simulink model "Simulator"  (R2024a)
settings: Solver=FixedStepAuto  StartTime=0.0  StopTime=1600  RelTol=1e-3
values from neighbouring files (symbols this model uses):
  T = loadturbineconstants('IEA15MW')    [init_controller.m]
  Wr0 = 0.60    (= 0.6)    [init_controller.m]
undefined symbols (not defined in the file or in its folder): DiscIntNeverNeededParam
libraries: DRC_SimulinkLibrary x3
settings Model: Creator=glazzerini  LastModifiedBy=glazzerini

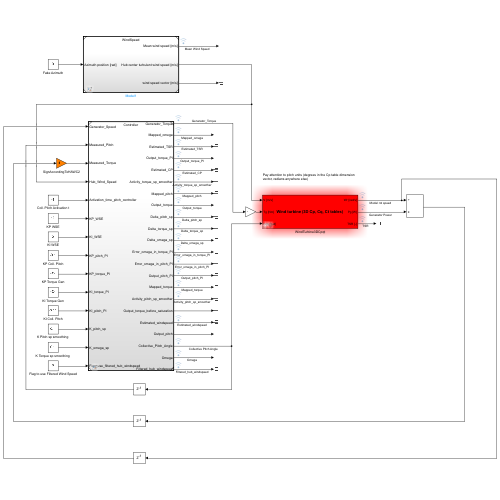
[thumbnail: Simulink's stored preview of the top-level diagram]
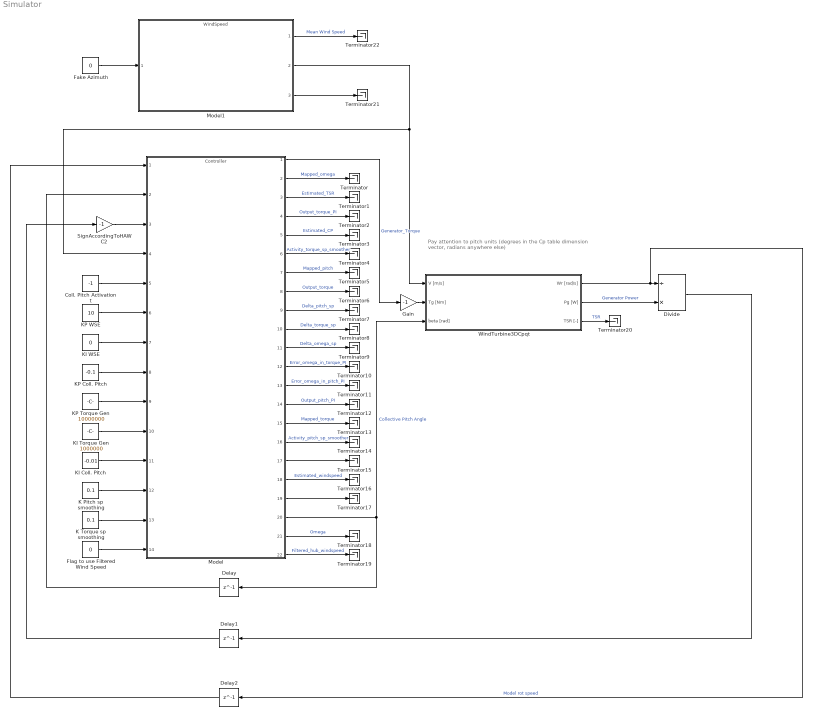
== system Simulator ==
  note: Pay attention to pitch units (degrees in the Cp table dimension vector, radians anywhere else)
  Coll. Pitch Activation t : Constant  Value=-1
  Delay : Delay  DelayLength=1
  Delay1 : Delay  DelayLength=1
  Delay2 : Delay  DelayLength=1
  Divide : Product  Inputs=/*
  Fake Azimuth : Constant  Value=0
  Flag to use Filtered Wind Speed : Constant  Value=0
  Gain : Gain  Gain=-1
  "K Pitch sp smoothing " : Constant  Value=0.1
  "K Torque sp smoothing " : Constant  Value=0.1
  KI Coll. Pitch : Constant  Value=-0.01
  KI Torque Gen : Constant  Value=1000000
  KI WSE : Constant  Value=0
  KP Coll. Pitch : Constant  Value=-0.1
  KP Torque Gen : Constant  Value=10000000
  KP WSE : Constant  Value=10
  Model : ModelReference  ModelNameDialog=Controller.slx  SimulationMode=Normal  ModelReferenceVersion=18.123
  Model1 : ModelReference  ModelNameDialog=WindSpeed.slx  SimulationMode=Normal  ModelReferenceVersion=9.19
  SignAccordingToHAWC2 : Gain  Gain=-1
  Terminator{,1..22} (23 alike) : Terminator
  WindTurbine3DCpqt : Subsystem  AncestorBlock=DRC_SimulinkLibrary/WindTurbine3DCpqt  mask{R=T.R, rho=T.rho, TMax=inf, JWr=T.Jlss, G=T.G, Wr0=Wr0, GenEfficiency=T.etag, CpArray=T.Cp, betaVec=deg2rad(T.CPitch), wsVec=T.CWindSpeed, omegaVec=T.COmega}
      mask prompts: R "Rotor radius [m]"; rho "Air density [kg/m^3]"; TMax "Maximum aerodynamic torque [Nm]"; JWr "Inertia low-speed shaft [kg m^2]"; G "Gearbox ratio [-]"; Wr0 "Rotor speed initial condition [rad/s]"; GenEfficiency "Generator Efficiency [-]"; CpArray "Cp matrix"; betaVec "Pitch vector [rad]"; wsVec "Wind speed vector [m/s]"; omegaVec "Omega vector [rad/s]"
      mask DialogControl CpGroupVar Prompt: Power coefficient (Cp)
      mask Display: disp('{\bf\fontsize{12}Wind turbine (3D Cp, Cq, Ct tables)}', 'texmode', 'on');
  wires:
  Model/1 -> Gain/1  "Generator_Torque"
  Model/20 -> WindTurbine3DCpqt/3(beta [rad]), Delay/1  "Collective Pitch Angle"
  WindTurbine3DCpqt/1(Wr [rad/s]) -> Divide/1, Delay2/1  "Model rot speed"
  Model/2 -> Terminator/1  "Mapped_omega"
  Model/3 -> Terminator1/1  "Estimated_TSR"
  Model/4 -> Terminator2/1  "Output_torque_PI"
  Model/5 -> Terminator3/1  "Estimated_CP"
  Model/6 -> Terminator4/1  "Activity_torque_sp_smoother"
  Model/7 -> Terminator5/1  "Mapped_pitch"
  Model/8 -> Terminator6/1  "Output_torque"
  Model/9 -> Terminator7/1  "Delta_pitch_sp"
  Model/10 -> Terminator8/1  "Delta_torque_sp"
  Model/11 -> Terminator9/1  "Delta_omega_sp"
  Model/12 -> Terminator10/1  "Error_omega_in_torque_PI"
  Model/13 -> Terminator11/1  "Error_omega_in_pitch_PI"
  Model/14 -> Terminator12/1  "Output_pitch_PI"
  Model/15 -> Terminator13/1  "Mapped_torque"
  Model/16 -> Terminator14/1  "Activity_pitch_sp_smoother"
  Model/17 -> Terminator15/1
  Model/18 -> Terminator16/1  "Estimated_windspeed"
  Model/19 -> Terminator17/1
  Model/21 -> Terminator18/1  "Omega"
  Model/22 -> Terminator19/1  "Filtered_hub_windspeed"
  Delay/1 -> Model/2
  WindTurbine3DCpqt/3(TSR [-]) -> Terminator20/1  "TSR"
  WindTurbine3DCpqt/2(Pg [W]) -> Divide/2  "Generator Power"
  Divide/1 -> Delay1/1
  Delay1/1 -> SignAccordingToHAWC2/1
  "K Torque sp smoothing "/1 -> Model/13
  "K Pitch sp smoothing "/1 -> Model/12
  Coll. Pitch Activation t/1 -> Model/5
  KP Torque Gen/1 -> Model/9
  KI Torque Gen/1 -> Model/10
  KP Coll. Pitch/1 -> Model/8
  KI Coll. Pitch/1 -> Model/11
  KP WSE/1 -> Model/6
  KI WSE/1 -> Model/7
  Model1/2 -> Model/4, WindTurbine3DCpqt/1(V [m/s])
  Fake Azimuth/1 -> Model1/1
  Model1/3 -> Terminator21/1
  Model1/1 -> Terminator22/1  "Mean Wind Speed"
  Gain/1 -> WindTurbine3DCpqt/2(Tg [Nm])
  Delay2/1 -> Model/1
  SignAccordingToHAWC2/1 -> Model/3
  Flag to use Filtered Wind Speed/1 -> Model/14

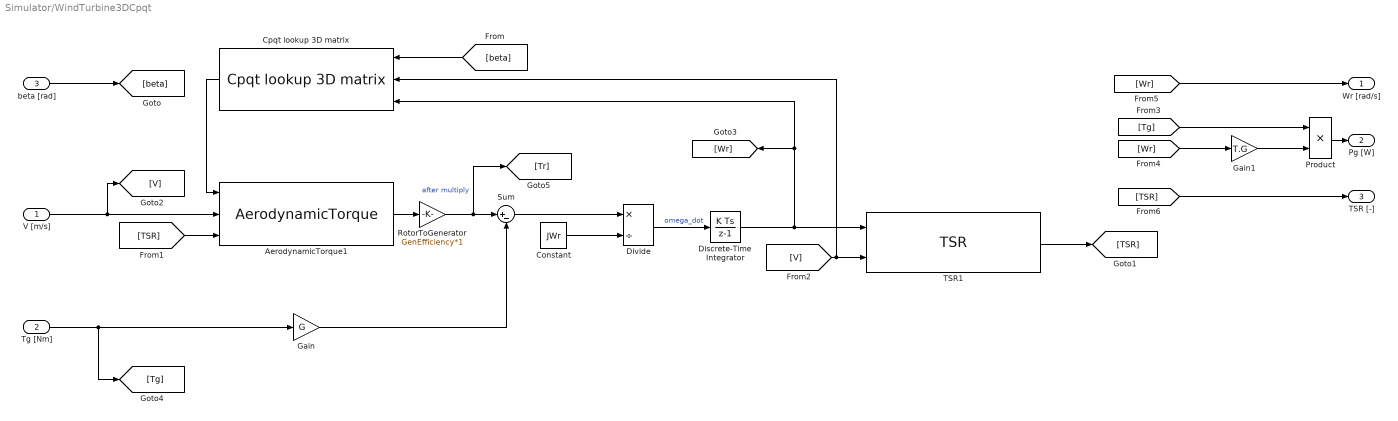
== system Simulator/WindTurbine3DCpqt ==
  V [m/s] : Inport
  Tg [Nm] : Inport  Port=2
  beta [rad] : Inport  Port=3
  AerodynamicTorque1 : DRC_SimulinkLibrary/AerodynamicTorque  R=R  rho=rho  TrMax=TMax
  Constant : Constant  Value=JWr
  Cpqt lookup 3D matrix : DRC_SimulinkLibrary/Cpqt lookup 3D matrix  CpqtGrid=CpArray  PitchVector=betaVec  WindSpeedVector=wsVec  OmegaVector=omegaVec
  Discrete-Time Integrator : DiscreteIntegrator  InitialCondition=Wr0  SampleTime=-1  ICPrevOutput=DiscIntNeverNeededParam  ICPrevScaledInput=DiscIntNeverNeededParam
  Divide : Product  Inputs=*/
  Gain : Gain  Gain=G
  Gain1 : Gain  Gain=T.G
  Product : Product
  RotorToGenerator : Gain  Gain=GenEfficiency*1
  Sum : Sum  Inputs=|+-
  TSR1 : DRC_SimulinkLibrary/TSR  RotorRadius=R
  Wr [rad/s] : Outport
  Pg [W] : Outport  Port=2
  TSR [-] : Outport  Port=3
  wires:
  Cpqt lookup 3D matrix/1 -> AerodynamicTorque1/1
  [TSR] -> TSR [-]/1
  [Wr] -> Wr [rad/s]/1
  [Tg] -> Product/1
  [Wr] -> Gain1/1
  Product/1 -> Pg [W]/1
  Gain1/1 -> Product/2
  [V] -> TSR1/2, Cpqt lookup 3D matrix/2
  TSR1/1 -> [TSR]
  Sum/1 -> Divide/1
  AerodynamicTorque1/1 -> RotorToGenerator/1
  Discrete-Time Integrator/1 -> TSR1/1, [Wr], Cpqt lookup 3D matrix/3
  Divide/1 -> Discrete-Time Integrator/1  "omega_dot"
  [beta] -> Cpqt lookup 3D matrix/1
  V [m/s]/1 -> AerodynamicTorque1/2, [V]
  Constant/1 -> Divide/2
  beta [rad]/1 -> [beta]
  Tg [Nm]/1 -> [Tg], Gain/1
  Gain/1 -> Sum/2
  [TSR] -> AerodynamicTorque1/3
  RotorToGenerator/1 -> Sum/1, [Tr]  "after multiply"
